simulink model "untitled"  (R2019a)
settings: Solver=FixedStepAuto  StartTime=0.0  StopTime=10  FixedStep=0.1  RelTol=1e-3
values from neighbouring files (symbols this model uses):
  a = 0.9    [lab10.m]
  b = 1.07    [lab10.m]
  c = 0.2773    [lab10.m]
  d = 0.0026    [lab10.m]
  g = 9.81    [lab10.m]
  Jw = 0.01    [lab10.m]
  mw = 1200    [lab10.m]
  rw = 0.3    [lab10.m]
  Tb = 0    [lab10.m]
settings Model: Creator=wojte  LastModifiedBy=wojte

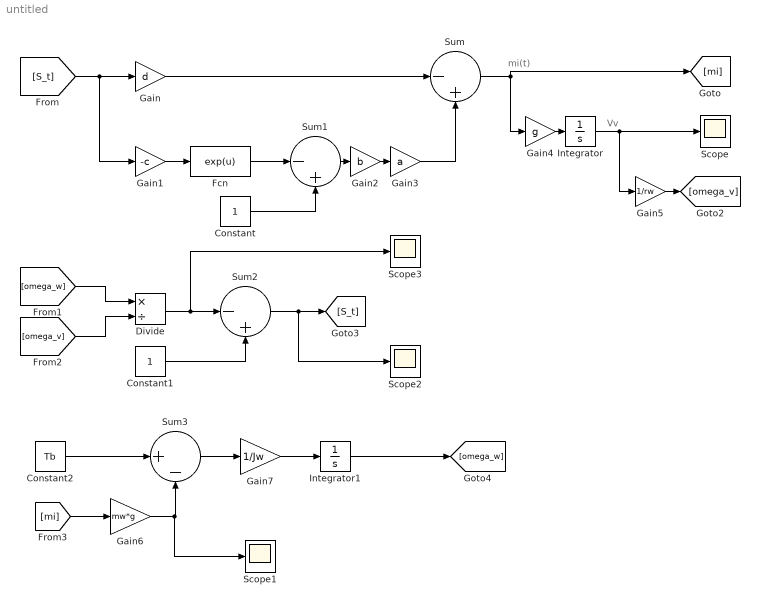
== system untitled ==
  note: Vv
  note: mi(t)
  Constant : Constant
  Constant1 : Constant
  Constant2 : Constant  Value=Tb
  Divide : Product  Inputs=*/
  Fcn : Fcn  Expr=exp(u)
  Gain : Gain  Gain=d
  Gain1 : Gain  Gain=-c
  Gain2 : Gain  Gain=b
  Gain3 : Gain  Gain=a
  Gain4 : Gain  Gain=g
  Gain5 : Gain  Gain=1/rw
  Gain6 : Gain  Gain=mw*g
  Gain7 : Gain  Gain=1/Jw
  Integrator : Integrator  InitialCondition=10
  Integrator1 : Integrator
  Scope{,1..3} (4 alike) : Scope
  Sum : Sum  Inputs=|-+
  Sum1 : Sum  Inputs=|-+
  Sum2 : Sum  Inputs=|-+
  Sum3 : Sum  Inputs=|+-
  wires:
  [S_t] -> Gain1/1, Gain/1
  Gain/1 -> Sum/1
  Gain1/1 -> Fcn/1
  Fcn/1 -> Sum1/1
  Constant/1 -> Sum1/2
  Sum1/1 -> Gain2/1
  Gain2/1 -> Gain3/1
  Gain3/1 -> Sum/2
  Sum/1 -> Gain4/1, [mi]
  Integrator/1 -> Scope/1, Gain5/1
  Gain4/1 -> Integrator/1
  Gain5/1 -> [omega_v]
  [omega_v] -> Divide/2
  [omega_w] -> Divide/1
  Divide/1 -> Scope3/1, Sum2/1
  Constant1/1 -> Sum2/2
  Sum2/1 -> Scope2/1, [S_t]
  Constant2/1 -> Sum3/1
  [mi] -> Gain6/1
  Gain6/1 -> Scope1/1, Sum3/2
  Sum3/1 -> Gain7/1
  Gain7/1 -> Integrator1/1
  Integrator1/1 -> [omega_w]
